simulink model "main"  (R2021b)
settings: Solver=VariableStepAuto  StartTime=0.0  StopTime=0.5  RelTol=1e-3
values from neighbouring files (symbols this model uses):
  Jt = 2*J0 + Ja2    (= 5.6e-06)    [comp.m]
  kc = 0.022    [comp.m]
  kcm = 1    [comp.m]
  kd = 0    [comp.m]
  ki = 389.9468    [comp.m]
  kp = 7.7989    [comp.m]
  ku = 0.022    [comp.m]
  La = 10e-6    (= 1e-05)    [comp.m]
  mr = 5e-3    (= 0.005)    [comp.m]
  Ra = 5.4    [comp.m]
libraries: simulink x1
settings Model: Creator=gaeta  LastModifiedBy=gaeta

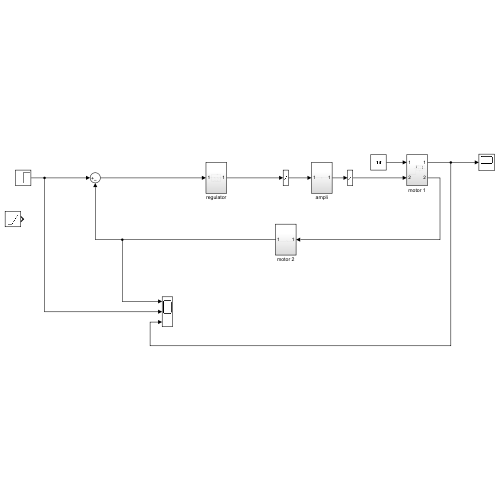
[thumbnail: Simulink's stored preview of the top-level diagram]
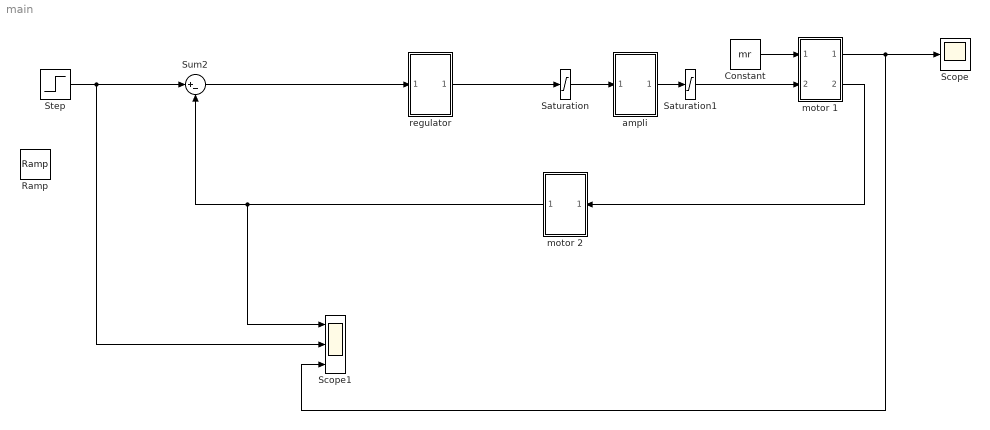
== system main ==
  Constant : Constant  Value=mr
  Ramp : simulink/Sources/Ramp  slope=2600*2*pi/60*ku/5  start=0  InitialOutput=0
  Saturation : Saturate  UpperLimit=15  LowerLimit=-15  ZeroCross=off
  Saturation1 : Saturate  UpperLimit=15  LowerLimit=-15  ZeroCross=off
  Scope : Scope
  Scope1 : Scope  NumInputPorts=3
  Step : Step  Time=0  After=2600*2*pi/60*ku  SampleTime=0
  Sum2 : Sum  Inputs=|+-
  ampli : Subsystem
  motor 1 : Subsystem
  motor 2 : Subsystem
  regulator : Subsystem
  wires:
  Sum2/1 -> regulator/1(In1)
  Constant/1 -> motor 1/1(In1)
  motor 1/1(Out1) -> Scope1/3, Scope/1
  regulator/1(Out1) -> Saturation/1
  ampli/1(Out1) -> Saturation1/1
  motor 1/2(Out2) -> motor 2/1(Vitesse mesurée en rad/sec)
  motor 2/1(Out1) -> Scope1/1, Sum2/2
  Saturation1/1 -> motor 1/2(In2)
  Saturation/1 -> ampli/1(In1)
  Step/1 -> Sum2/1, Scope1/2

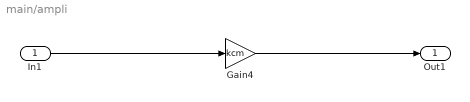
== system main/ampli ==
  In1 : Inport
  Gain4 : Gain  Gain=kcm
  Out1 : Outport
  wires:
  Gain4/1 -> Out1/1
  In1/1 -> Gain4/1

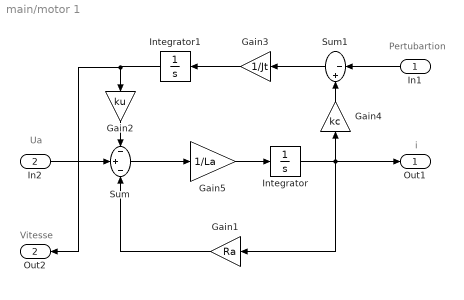
== system main/motor 1 ==
  note: i
  note: Pertubartion
  note: Vitesse
  note: Ua
  In1 : Inport
  In2 : Inport  Port=2
  Gain1 : Gain  Gain=Ra
  Gain2 : Gain  Gain=ku
  Gain3 : Gain  Gain=1/Jt
  Gain4 : Gain  Gain=kc
  Gain5 : Gain  Gain=1/La
  Integrator : Integrator  LimitOutput=on  UpperSaturationLimit=2  LowerSaturationLimit=-2
  Integrator1 : Integrator
  Sum : Sum  Inputs=-+-
  Sum1 : Sum  Inputs=|-+
  Out1 : Outport
  Out2 : Outport  Port=2
  wires:
  Gain5/1 -> Integrator/1
  Gain1/1 -> Sum/3
  Sum/1 -> Gain5/1
  Sum1/1 -> Gain3/1
  Integrator/1 -> Gain4/1, Out1/1, Gain1/1
  In2/1 -> Sum/2
  Integrator1/1 -> Out2/1, Gain2/1
  Gain2/1 -> Sum/1
  Gain3/1 -> Integrator1/1
  In1/1 -> Sum1/1
  Gain4/1 -> Sum1/2

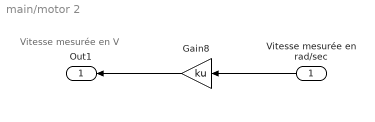
== system main/motor 2 ==
  note: Vitesse mesurée en V
  Vitesse mesurée en rad/sec : Inport
  Gain8 : Gain  Gain=ku
  Out1 : Outport
  wires:
  Vitesse mesurée en rad/sec/1 -> Gain8/1
  Gain8/1 -> Out1/1

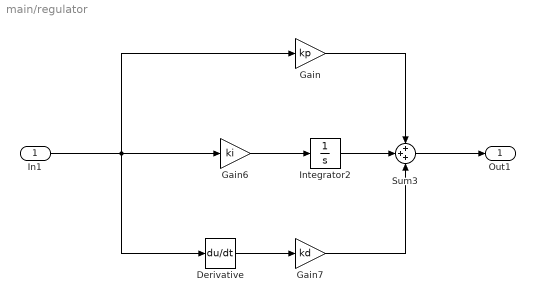
== system main/regulator ==
  In1 : Inport
  Derivative : Derivative
  Gain : Gain  Gain=kp
  Gain6 : Gain  Gain=ki
  Gain7 : Gain  Gain=kd
  Integrator2 : Integrator  LimitOutput=on  UpperSaturationLimit=15  LowerSaturationLimit=-15
  Sum3 : Sum  Inputs=+++
  Out1 : Outport
  wires:
  Gain/1 -> Sum3/1
  Sum3/1 -> Out1/1
  In1/1 -> Gain6/1, Derivative/1, Gain/1
  Integrator2/1 -> Sum3/2
  Derivative/1 -> Gain7/1
  Gain6/1 -> Integrator2/1
  Gain7/1 -> Sum3/3
